simulink model "IEEE5BusSystemModel_std_UFLS"  (R2019b)
settings: Solver=ode4  StartTime=0.0  StopTime=300  MaxStep=1e-4  RelTol=1e-3
InitFcn:
  | startup_RTS
values from neighbouring files (symbols this model uses):
  C = b/(2*pi*60*Zn)    [startup_RTS.m]
  C0 = C/3    [startup_RTS.m]
  fn = 50    [startup_RTS.m]
  In = Sn/(sqrt(3)*Vn)    [startup_RTS.m]
  L = x*Zn/(2*pi*60)    [startup_RTS.m]
  L0 = 3*L    [startup_RTS.m]
  len = ceil(0.95*300000*T_prop)    [startup_RTS.m]
  PL1 = 300e6    (= 300000000)    [startup_RTS.m]
  PL2 = 300e6    (= 300000000)    [startup_RTS.m]
  PL3 = 300e6    (= 300000000)    [startup_RTS.m]
  QL1 = 30e6    (= 30000000)    [startup_RTS.m]
  QL2 = 30e6    (= 30000000)    [startup_RTS.m]
  QL3 = 30e6    (= 30000000)    [startup_RTS.m]
  R = r*Zn    [startup_RTS.m]
  R0 = 3*R    [startup_RTS.m]
  Sn = 1000e6    (= 1000000000)    [startup_RTS.m]
  t_cont = 100    [startup_RTS.m]
  Vn = 345e3    (= 345000)    [startup_RTS.m]
undefined symbols (not defined in the file or in its folder): D1, Delta
libraries: powerlib x42, powerlib_meascontrol x39, dspswit3 x10, dspstat3 x3, sps_avr x3, spsExcitationSystemModel x3
(part 3 of 7)

== system IEEE5BusSystemModel_std_UFLS/Subsystem2/PMU_e-IpDFT_P-class ==
  Uabc : Inport
  Constant1 : Constant  Value=dF  SampleTime=Ts_p
  Constant2 : Constant  Value=0  SampleTime=Ts_p
  Counter : dspswit3/Counter  Direction=Up  CountEvent=Free running  CounterSize=User defined  MaxCount=M-1  InitialCount=1  Output=Hit  HitValue=0  ResetInput=off  SamplesPerFrame=1  Ts=Ts_p  CntDtype=double  HitDtype=Logical
  Demux1 : Demux  Outputs=3
  Ia_est : Subsystem
  Terminator3 : Terminator
  Terminator4 : Terminator
  Frequency : Outport  VectorParamsAs1DForOutWhenUnconnected=off
  Amplitude : Outport  Port=2  VectorParamsAs1DForOutWhenUnconnected=off
  Phase : Outport  Port=3  VectorParamsAs1DForOutWhenUnconnected=off
  wires:
  Ia_est/1(Frequency) -> Frequency/1
  Ia_est/2(Amplitude) -> Amplitude/1
  Ia_est/3(Phase) -> Phase/1
  Uabc/1 -> Demux1/1
  Demux1/1 -> Ia_est/1(signal)
  Counter/1 -> Ia_est/2(Hit)
  Constant1/1 -> Ia_est/4(dF [Hz])
  Constant2/1 -> Ia_est/3(dT [s])
  Demux1/2 -> Terminator3/1
  Demux1/3 -> Terminator4/1

== system IEEE5BusSystemModel_std_UFLS/Subsystem2/PMU_e-IpDFT_P-class1 ==
  Uabc : Inport
  Constant1 : Constant  Value=dF  SampleTime=Ts_p
  Constant2 : Constant  Value=0  SampleTime=Ts_p
  Counter : dspswit3/Counter  Direction=Up  CountEvent=Free running  CounterSize=User defined  MaxCount=M-1  InitialCount=1  Output=Hit  HitValue=0  ResetInput=off  SamplesPerFrame=1  Ts=Ts_p  CntDtype=double  HitDtype=Logical
  Demux1 : Demux  Outputs=3
  Ia_est : Subsystem
  Terminator3 : Terminator
  Terminator4 : Terminator
  Frequency : Outport  VectorParamsAs1DForOutWhenUnconnected=off
  Amplitude : Outport  Port=2  VectorParamsAs1DForOutWhenUnconnected=off
  Phase : Outport  Port=3  VectorParamsAs1DForOutWhenUnconnected=off
  wires:
  Demux1/3 -> Terminator4/1
  Demux1/2 -> Terminator3/1
  Constant2/1 -> Ia_est/3(dT [s])
  Constant1/1 -> Ia_est/4(dF [Hz])
  Counter/1 -> Ia_est/2(Hit)
  Demux1/1 -> Ia_est/1(signal)
  Uabc/1 -> Demux1/1
  Ia_est/3(Phase) -> Phase/1
  Ia_est/2(Amplitude) -> Amplitude/1
  Ia_est/1(Frequency) -> Frequency/1

== system IEEE5BusSystemModel_std_UFLS/Subsystem3/PMU_e-IpDFT_P-class ==
  Uabc : Inport
  Constant1 : Constant  Value=dF  SampleTime=Ts_p
  Constant2 : Constant  Value=0  SampleTime=Ts_p
  Counter : dspswit3/Counter  Direction=Up  CountEvent=Free running  CounterSize=User defined  MaxCount=M-1  InitialCount=1  Output=Hit  HitValue=0  ResetInput=off  SamplesPerFrame=1  Ts=Ts_p  CntDtype=double  HitDtype=Logical
  Demux1 : Demux  Outputs=3
  Ia_est : Subsystem
  Terminator3 : Terminator
  Terminator4 : Terminator
  Frequency : Outport  VectorParamsAs1DForOutWhenUnconnected=off
  Amplitude : Outport  Port=2  VectorParamsAs1DForOutWhenUnconnected=off
  Phase : Outport  Port=3  VectorParamsAs1DForOutWhenUnconnected=off
  wires:
  Demux1/3 -> Terminator4/1
  Demux1/2 -> Terminator3/1
  Constant2/1 -> Ia_est/3(dT [s])
  Constant1/1 -> Ia_est/4(dF [Hz])
  Counter/1 -> Ia_est/2(Hit)
  Demux1/1 -> Ia_est/1(signal)
  Uabc/1 -> Demux1/1
  Ia_est/3(Phase) -> Phase/1
  Ia_est/2(Amplitude) -> Amplitude/1
  Ia_est/1(Frequency) -> Frequency/1

== system IEEE5BusSystemModel_std_UFLS/Subsystem3/PMU_e-IpDFT_P-class1 ==
  Uabc : Inport
  Constant1 : Constant  Value=dF  SampleTime=Ts_p
  Constant2 : Constant  Value=0  SampleTime=Ts_p
  Counter : dspswit3/Counter  Direction=Up  CountEvent=Free running  CounterSize=User defined  MaxCount=M-1  InitialCount=1  Output=Hit  HitValue=0  ResetInput=off  SamplesPerFrame=1  Ts=Ts_p  CntDtype=double  HitDtype=Logical
  Demux1 : Demux  Outputs=3
  Ia_est : Subsystem
  Terminator3 : Terminator
  Terminator4 : Terminator
  Frequency : Outport  VectorParamsAs1DForOutWhenUnconnected=off
  Amplitude : Outport  Port=2  VectorParamsAs1DForOutWhenUnconnected=off
  Phase : Outport  Port=3  VectorParamsAs1DForOutWhenUnconnected=off
  wires:
  Ia_est/1(Frequency) -> Frequency/1
  Ia_est/2(Amplitude) -> Amplitude/1
  Ia_est/3(Phase) -> Phase/1
  Uabc/1 -> Demux1/1
  Demux1/1 -> Ia_est/1(signal)
  Counter/1 -> Ia_est/2(Hit)
  Constant1/1 -> Ia_est/4(dF [Hz])
  Constant2/1 -> Ia_est/3(dT [s])
  Demux1/2 -> Terminator3/1
  Demux1/3 -> Terminator4/1

== system IEEE5BusSystemModel_std_UFLS/Subsystem4/PMU_e-IpDFT_P-class ==
  Uabc : Inport
  Constant1 : Constant  Value=dF  SampleTime=Ts_p
  Constant2 : Constant  Value=0  SampleTime=Ts_p
  Counter : dspswit3/Counter  Direction=Up  CountEvent=Free running  CounterSize=User defined  MaxCount=M-1  InitialCount=1  Output=Hit  HitValue=0  ResetInput=off  SamplesPerFrame=1  Ts=Ts_p  CntDtype=double  HitDtype=Logical
  Demux1 : Demux  Outputs=3
  Ia_est : Subsystem
  Terminator3 : Terminator
  Terminator4 : Terminator
  Frequency : Outport  VectorParamsAs1DForOutWhenUnconnected=off
  Amplitude : Outport  Port=2  VectorParamsAs1DForOutWhenUnconnected=off
  Phase : Outport  Port=3  VectorParamsAs1DForOutWhenUnconnected=off
  wires:
  Ia_est/1(Frequency) -> Frequency/1
  Ia_est/2(Amplitude) -> Amplitude/1
  Ia_est/3(Phase) -> Phase/1
  Uabc/1 -> Demux1/1
  Demux1/1 -> Ia_est/1(signal)
  Counter/1 -> Ia_est/2(Hit)
  Constant1/1 -> Ia_est/4(dF [Hz])
  Constant2/1 -> Ia_est/3(dT [s])
  Demux1/2 -> Terminator3/1
  Demux1/3 -> Terminator4/1

== system IEEE5BusSystemModel_std_UFLS/Subsystem4/PMU_e-IpDFT_P-class1 ==
  Uabc : Inport
  Constant1 : Constant  Value=dF  SampleTime=Ts_p
  Constant2 : Constant  Value=0  SampleTime=Ts_p
  Counter : dspswit3/Counter  Direction=Up  CountEvent=Free running  CounterSize=User defined  MaxCount=M-1  InitialCount=1  Output=Hit  HitValue=0  ResetInput=off  SamplesPerFrame=1  Ts=Ts_p  CntDtype=double  HitDtype=Logical
  Demux1 : Demux  Outputs=3
  Ia_est : Subsystem
  Terminator3 : Terminator
  Terminator4 : Terminator
  Frequency : Outport  VectorParamsAs1DForOutWhenUnconnected=off
  Amplitude : Outport  Port=2  VectorParamsAs1DForOutWhenUnconnected=off
  Phase : Outport  Port=3  VectorParamsAs1DForOutWhenUnconnected=off
  wires:
  Demux1/3 -> Terminator4/1
  Demux1/2 -> Terminator3/1
  Constant2/1 -> Ia_est/3(dT [s])
  Constant1/1 -> Ia_est/4(dF [Hz])
  Counter/1 -> Ia_est/2(Hit)
  Demux1/1 -> Ia_est/1(signal)
  Uabc/1 -> Demux1/1
  Ia_est/3(Phase) -> Phase/1
  Ia_est/2(Amplitude) -> Amplitude/1
  Ia_est/1(Frequency) -> Frequency/1

== system IEEE5BusSystemModel_std_UFLS/Subsystem5/PMU_e-IpDFT_P-class ==
  Uabc : Inport
  Constant1 : Constant  Value=dF  SampleTime=Ts_p
  Constant2 : Constant  Value=0  SampleTime=Ts_p
  Counter : dspswit3/Counter  Direction=Up  CountEvent=Free running  CounterSize=User defined  MaxCount=M-1  InitialCount=1  Output=Hit  HitValue=0  ResetInput=off  SamplesPerFrame=1  Ts=Ts_p  CntDtype=double  HitDtype=Logical
  Demux1 : Demux  Outputs=3
  Ia_est : Subsystem
  Terminator3 : Terminator
  Terminator4 : Terminator
  Frequency : Outport  VectorParamsAs1DForOutWhenUnconnected=off
  Amplitude : Outport  Port=2  VectorParamsAs1DForOutWhenUnconnected=off
  Phase : Outport  Port=3  VectorParamsAs1DForOutWhenUnconnected=off
  wires:
  Ia_est/1(Frequency) -> Frequency/1
  Ia_est/2(Amplitude) -> Amplitude/1
  Ia_est/3(Phase) -> Phase/1
  Uabc/1 -> Demux1/1
  Demux1/1 -> Ia_est/1(signal)
  Counter/1 -> Ia_est/2(Hit)
  Constant1/1 -> Ia_est/4(dF [Hz])
  Constant2/1 -> Ia_est/3(dT [s])
  Demux1/2 -> Terminator3/1
  Demux1/3 -> Terminator4/1

== system IEEE5BusSystemModel_std_UFLS/Subsystem5/PMU_e-IpDFT_P-class1 ==
  Uabc : Inport
  Constant1 : Constant  Value=dF  SampleTime=Ts_p
  Constant2 : Constant  Value=0  SampleTime=Ts_p
  Counter : dspswit3/Counter  Direction=Up  CountEvent=Free running  CounterSize=User defined  MaxCount=M-1  InitialCount=1  Output=Hit  HitValue=0  ResetInput=off  SamplesPerFrame=1  Ts=Ts_p  CntDtype=double  HitDtype=Logical
  Demux1 : Demux  Outputs=3
  Ia_est : Subsystem
  Terminator3 : Terminator
  Terminator4 : Terminator
  Frequency : Outport  VectorParamsAs1DForOutWhenUnconnected=off
  Amplitude : Outport  Port=2  VectorParamsAs1DForOutWhenUnconnected=off
  Phase : Outport  Port=3  VectorParamsAs1DForOutWhenUnconnected=off
  wires:
  Demux1/3 -> Terminator4/1
  Demux1/2 -> Terminator3/1
  Constant2/1 -> Ia_est/3(dT [s])
  Constant1/1 -> Ia_est/4(dF [Hz])
  Counter/1 -> Ia_est/2(Hit)
  Demux1/1 -> Ia_est/1(signal)
  Uabc/1 -> Demux1/1
  Ia_est/3(Phase) -> Phase/1
  Ia_est/2(Amplitude) -> Amplitude/1
  Ia_est/1(Frequency) -> Frequency/1

== system IEEE5BusSystemModel_std_UFLS/Dynamic Load/Load 8/Load shedding ==
  note: P=P0(V/V0) Kpv * [1+Kpf(f-f0)]
  note: Q=Q0(V/V0)[Kqv(1+Kqf(f-f0)]
  note: Q=Q0(V/V0)[Kqv(1+Kqf(f-f0)]
  note: P=P0(V/V0) Kpv * [1+Kpf(f-f0)]
  " f_PLL" : Inport
  Vamp_rms : Inport  Port=2
  load : Inport  Port=3
  Constant2 : Constant
  Constant3 : Constant  Value=50
  Constant4 : Constant
  Demux : Demux  Outputs=2
  Kpf : Gain
  Kpv : Constant  Value=1.4
  Kqf : Gain  Gain=-1.4
  Kqv : Constant  Value=1.5
  Math Function : Math  Operator=pow  SaturateOnIntegerOverflow=on
  Math Function1 : Math  Operator=pow  SaturateOnIntegerOverflow=on
  Mux : Mux  Inputs=2
  Product2 : Product  Inputs=3
  Product4 : Product  Inputs=3
  Saturation : Saturate  UpperLimit=1.2  LowerLimit=0
  Saturation1 : Saturate  UpperLimit=3/fn  LowerLimit=-3/fn
  Sum : Sum  Inputs=|++
  Sum1 : Sum  Inputs=|+-
  Sum2 : Sum  Inputs=|++
  V/V0 : Gain  Gain=sqrt(3)/345e3
  fpu : Gain  Gain=0.02
  Load Power : Outport  VectorParamsAs1DForOutWhenUnconnected=off
  wires:
  Product2/1 -> Mux/1
  Demux/1 -> Product2/1  "P0"
  Math Function/1 -> Product2/2
  Sum/1 -> Product2/3
  Constant2/1 -> Sum/1
  Constant3/1 -> Sum1/2
  Demux/2 -> Product4/1  "Q0"
  Math Function1/1 -> Product4/2
  Sum2/1 -> Product4/3
  Constant4/1 -> Sum2/1
  Sum1/1 -> fpu/1
  Product4/1 -> Mux/2
  Saturation1/1 -> Kpf/1, Kqf/1
  load/1 -> Demux/1
  fpu/1 -> Saturation1/1
  " f_PLL"/1 -> Sum1/1
  Vamp_rms/1 -> V/V0/1
  Mux/1 -> Load Power/1
  V/V0/1 -> Saturation/1  "Vamp-p"
  Saturation/1 -> Math Function/1, Math Function1/1
  Kpv/1 -> Math Function/2
  Kqv/1 -> Math Function1/2
  Kqf/1 -> Sum2/2
  Kpf/1 -> Sum/2

== system IEEE5BusSystemModel_std_UFLS/Dynamic Load1/Load 8/Load shedding ==
  note: P=P0(V/V0) Kpv * [1+Kpf(f-f0)]
  note: Q=Q0(V/V0)[Kqv(1+Kqf(f-f0)]
  note: Q=Q0(V/V0)[Kqv(1+Kqf(f-f0)]
  note: P=P0(V/V0) Kpv * [1+Kpf(f-f0)]
  " f_PLL" : Inport
  Vamp_rms : Inport  Port=2
  load : Inport  Port=3
  Constant2 : Constant
  Constant3 : Constant  Value=50
  Constant4 : Constant
  Demux : Demux  Outputs=2
  Kpf : Gain
  Kpv : Constant  Value=1.4
  Kqf : Gain  Gain=-1.6
  Kqv : Constant  Value=1.7
  Math Function : Math  Operator=pow  SaturateOnIntegerOverflow=on
  Math Function1 : Math  Operator=pow  SaturateOnIntegerOverflow=on
  Mux : Mux  Inputs=2
  Product2 : Product  Inputs=3
  Product4 : Product  Inputs=3
  Saturation : Saturate  UpperLimit=1.2  LowerLimit=0
  Saturation1 : Saturate  UpperLimit=3/fn  LowerLimit=-3/fn
  Sum : Sum  Inputs=|++
  Sum1 : Sum  Inputs=|+-
  Sum2 : Sum  Inputs=|++
  V/V0 : Gain  Gain=sqrt(3)/345e3
  fpu : Gain  Gain=0.02
  Load Power : Outport  VectorParamsAs1DForOutWhenUnconnected=off
  wires:
  Kpf/1 -> Sum/2
  Kqf/1 -> Sum2/2
  Kqv/1 -> Math Function1/2
  Kpv/1 -> Math Function/2
  Saturation/1 -> Math Function1/1, Math Function/1
  V/V0/1 -> Saturation/1  "Vamp-p"
  Mux/1 -> Load Power/1
  Vamp_rms/1 -> V/V0/1
  " f_PLL"/1 -> Sum1/1
  fpu/1 -> Saturation1/1
  load/1 -> Demux/1
  Saturation1/1 -> Kqf/1, Kpf/1
  Product4/1 -> Mux/2
  Sum1/1 -> fpu/1
  Constant4/1 -> Sum2/1
  Sum2/1 -> Product4/3
  Math Function1/1 -> Product4/2
  Demux/2 -> Product4/1  "Q0"
  Constant3/1 -> Sum1/2
  Constant2/1 -> Sum/1
  Sum/1 -> Product2/3
  Math Function/1 -> Product2/2
  Demux/1 -> Product2/1  "P0"
  Product2/1 -> Mux/1

== system IEEE5BusSystemModel_std_UFLS/Dynamic Load2/Load 8/Load shedding ==
  note: P=P0(V/V0) Kpv * [1+Kpf(f-f0)]
  note: Q=Q0(V/V0)[Kqv(1+Kqf(f-f0)]
  note: Q=Q0(V/V0)[Kqv(1+Kqf(f-f0)]
  note: P=P0(V/V0) Kpv * [1+Kpf(f-f0)]
  " f_PLL" : Inport
  Vamp_rms : Inport  Port=2
  load : Inport  Port=3
  Constant2 : Constant
  Constant3 : Constant  Value=50
  Constant4 : Constant
  Demux : Demux  Outputs=2
  Kpf : Gain
  Kpv : Constant  Value=1.5
  Kqf : Gain  Gain=-1.5
  Kqv : Constant  Value=1.9
  Math Function : Math  Operator=pow  SaturateOnIntegerOverflow=on
  Math Function1 : Math  Operator=pow  SaturateOnIntegerOverflow=on
  Mux : Mux  Inputs=2
  Product2 : Product  Inputs=3
  Product4 : Product  Inputs=3
  Saturation : Saturate  UpperLimit=1.2  LowerLimit=0
  Saturation1 : Saturate  UpperLimit=3/fn  LowerLimit=-3/fn
  Sum : Sum  Inputs=|++
  Sum1 : Sum  Inputs=|+-
  Sum2 : Sum  Inputs=|++
  V/V0 : Gain  Gain=sqrt(3)/345e3
  fpu : Gain  Gain=0.02
  Load Power : Outport  VectorParamsAs1DForOutWhenUnconnected=off
  wires:
  Product2/1 -> Mux/1
  Demux/1 -> Product2/1  "P0"
  Math Function/1 -> Product2/2
  Sum/1 -> Product2/3
  Constant2/1 -> Sum/1
  Constant3/1 -> Sum1/2
  Demux/2 -> Product4/1  "Q0"
  Math Function1/1 -> Product4/2
  Sum2/1 -> Product4/3
  Constant4/1 -> Sum2/1
  Sum1/1 -> fpu/1
  Product4/1 -> Mux/2
  Saturation1/1 -> Kpf/1, Kqf/1
  load/1 -> Demux/1
  fpu/1 -> Saturation1/1
  " f_PLL"/1 -> Sum1/1
  Vamp_rms/1 -> V/V0/1
  Mux/1 -> Load Power/1
  V/V0/1 -> Saturation/1  "Vamp-p"
  Saturation/1 -> Math Function/1, Math Function1/1
  Kpv/1 -> Math Function/2
  Kqv/1 -> Math Function1/2
  Kqf/1 -> Sum2/2
  Kpf/1 -> Sum/2

== system IEEE5BusSystemModel_std_UFLS/Subsystem1/PMU_e-IpDFT_P-class/Ia_est ==
  signal : Inport
  Hit : Inport  Port=2
  dT [s] : Inport  Port=3
  dF [Hz] : Inport  Port=4
  Synchrophasor estimation : Subsystem
  mSDFT : Subsystem
  Frequency : Outport  VectorParamsAs1DForOutWhenUnconnected=off
  Amplitude : Outport  Port=2  VectorParamsAs1DForOutWhenUnconnected=off
  Phase : Outport  Port=3  VectorParamsAs1DForOutWhenUnconnected=off
  wires:
  dT [s]/1 -> Synchrophasor estimation/2(dT [s])
  Hit/1 -> mSDFT/2(Hit)
  Synchrophasor estimation/3(Phase) -> Phase/1
  Synchrophasor estimation/2(Amplitude) -> Amplitude/1
  mSDFT/1(DFT) -> Synchrophasor estimation/1(DFT)
  signal/1 -> mSDFT/1(signal)
  Synchrophasor estimation/1(Frequency) -> Frequency/1
  dF [Hz]/1 -> Synchrophasor estimation/3(dF [Hz])

== system IEEE5BusSystemModel_std_UFLS/Subsystem1/PMU_e-IpDFT_P-class1/Ia_est ==
  signal : Inport
  Hit : Inport  Port=2
  dT [s] : Inport  Port=3
  dF [Hz] : Inport  Port=4
  Synchrophasor estimation : Subsystem
  mSDFT : Subsystem
  Frequency : Outport  VectorParamsAs1DForOutWhenUnconnected=off
  Amplitude : Outport  Port=2  VectorParamsAs1DForOutWhenUnconnected=off
  Phase : Outport  Port=3  VectorParamsAs1DForOutWhenUnconnected=off
  wires:
  dF [Hz]/1 -> Synchrophasor estimation/3(dF [Hz])
  Synchrophasor estimation/1(Frequency) -> Frequency/1
  signal/1 -> mSDFT/1(signal)
  mSDFT/1(DFT) -> Synchrophasor estimation/1(DFT)
  Synchrophasor estimation/2(Amplitude) -> Amplitude/1
  Synchrophasor estimation/3(Phase) -> Phase/1
  Hit/1 -> mSDFT/2(Hit)
  dT [s]/1 -> Synchrophasor estimation/2(dT [s])

== system IEEE5BusSystemModel_std_UFLS/Subsystem2/PMU_e-IpDFT_P-class/Ia_est ==
  signal : Inport
  Hit : Inport  Port=2
  dT [s] : Inport  Port=3
  dF [Hz] : Inport  Port=4
  Synchrophasor estimation : Subsystem
  mSDFT : Subsystem
  Frequency : Outport  VectorParamsAs1DForOutWhenUnconnected=off
  Amplitude : Outport  Port=2  VectorParamsAs1DForOutWhenUnconnected=off
  Phase : Outport  Port=3  VectorParamsAs1DForOutWhenUnconnected=off
  wires:
  dF [Hz]/1 -> Synchrophasor estimation/3(dF [Hz])
  Synchrophasor estimation/1(Frequency) -> Frequency/1
  signal/1 -> mSDFT/1(signal)
  mSDFT/1(DFT) -> Synchrophasor estimation/1(DFT)
  Synchrophasor estimation/2(Amplitude) -> Amplitude/1
  Synchrophasor estimation/3(Phase) -> Phase/1
  Hit/1 -> mSDFT/2(Hit)
  dT [s]/1 -> Synchrophasor estimation/2(dT [s])

== system IEEE5BusSystemModel_std_UFLS/Subsystem2/PMU_e-IpDFT_P-class1/Ia_est ==
  signal : Inport
  Hit : Inport  Port=2
  dT [s] : Inport  Port=3
  dF [Hz] : Inport  Port=4
  Synchrophasor estimation : Subsystem
  mSDFT : Subsystem
  Frequency : Outport  VectorParamsAs1DForOutWhenUnconnected=off
  Amplitude : Outport  Port=2  VectorParamsAs1DForOutWhenUnconnected=off
  Phase : Outport  Port=3  VectorParamsAs1DForOutWhenUnconnected=off
  wires:
  dT [s]/1 -> Synchrophasor estimation/2(dT [s])
  Hit/1 -> mSDFT/2(Hit)
  Synchrophasor estimation/3(Phase) -> Phase/1
  Synchrophasor estimation/2(Amplitude) -> Amplitude/1
  mSDFT/1(DFT) -> Synchrophasor estimation/1(DFT)
  signal/1 -> mSDFT/1(signal)
  Synchrophasor estimation/1(Frequency) -> Frequency/1
  dF [Hz]/1 -> Synchrophasor estimation/3(dF [Hz])

== system IEEE5BusSystemModel_std_UFLS/Subsystem3/PMU_e-IpDFT_P-class/Ia_est ==
  signal : Inport
  Hit : Inport  Port=2
  dT [s] : Inport  Port=3
  dF [Hz] : Inport  Port=4
  Synchrophasor estimation : Subsystem
  mSDFT : Subsystem
  Frequency : Outport  VectorParamsAs1DForOutWhenUnconnected=off
  Amplitude : Outport  Port=2  VectorParamsAs1DForOutWhenUnconnected=off
  Phase : Outport  Port=3  VectorParamsAs1DForOutWhenUnconnected=off
  wires:
  dT [s]/1 -> Synchrophasor estimation/2(dT [s])
  Hit/1 -> mSDFT/2(Hit)
  Synchrophasor estimation/3(Phase) -> Phase/1
  Synchrophasor estimation/2(Amplitude) -> Amplitude/1
  mSDFT/1(DFT) -> Synchrophasor estimation/1(DFT)
  signal/1 -> mSDFT/1(signal)
  Synchrophasor estimation/1(Frequency) -> Frequency/1
  dF [Hz]/1 -> Synchrophasor estimation/3(dF [Hz])

== system IEEE5BusSystemModel_std_UFLS/Subsystem3/PMU_e-IpDFT_P-class1/Ia_est ==
  signal : Inport
  Hit : Inport  Port=2
  dT [s] : Inport  Port=3
  dF [Hz] : Inport  Port=4
  Synchrophasor estimation : Subsystem
  mSDFT : Subsystem
  Frequency : Outport  VectorParamsAs1DForOutWhenUnconnected=off
  Amplitude : Outport  Port=2  VectorParamsAs1DForOutWhenUnconnected=off
  Phase : Outport  Port=3  VectorParamsAs1DForOutWhenUnconnected=off
  wires:
  dF [Hz]/1 -> Synchrophasor estimation/3(dF [Hz])
  Synchrophasor estimation/1(Frequency) -> Frequency/1
  signal/1 -> mSDFT/1(signal)
  mSDFT/1(DFT) -> Synchrophasor estimation/1(DFT)
  Synchrophasor estimation/2(Amplitude) -> Amplitude/1
  Synchrophasor estimation/3(Phase) -> Phase/1
  Hit/1 -> mSDFT/2(Hit)
  dT [s]/1 -> Synchrophasor estimation/2(dT [s])

== system IEEE5BusSystemModel_std_UFLS/Subsystem4/PMU_e-IpDFT_P-class/Ia_est ==
  signal : Inport
  Hit : Inport  Port=2
  dT [s] : Inport  Port=3
  dF [Hz] : Inport  Port=4
  Synchrophasor estimation : Subsystem
  mSDFT : Subsystem
  Frequency : Outport  VectorParamsAs1DForOutWhenUnconnected=off
  Amplitude : Outport  Port=2  VectorParamsAs1DForOutWhenUnconnected=off
  Phase : Outport  Port=3  VectorParamsAs1DForOutWhenUnconnected=off
  wires:
  dF [Hz]/1 -> Synchrophasor estimation/3(dF [Hz])
  Synchrophasor estimation/1(Frequency) -> Frequency/1
  signal/1 -> mSDFT/1(signal)
  mSDFT/1(DFT) -> Synchrophasor estimation/1(DFT)
  Synchrophasor estimation/2(Amplitude) -> Amplitude/1
  Synchrophasor estimation/3(Phase) -> Phase/1
  Hit/1 -> mSDFT/2(Hit)
  dT [s]/1 -> Synchrophasor estimation/2(dT [s])

== system IEEE5BusSystemModel_std_UFLS/Subsystem4/PMU_e-IpDFT_P-class1/Ia_est ==
  signal : Inport
  Hit : Inport  Port=2
  dT [s] : Inport  Port=3
  dF [Hz] : Inport  Port=4
  Synchrophasor estimation : Subsystem
  mSDFT : Subsystem
  Frequency : Outport  VectorParamsAs1DForOutWhenUnconnected=off
  Amplitude : Outport  Port=2  VectorParamsAs1DForOutWhenUnconnected=off
  Phase : Outport  Port=3  VectorParamsAs1DForOutWhenUnconnected=off
  wires:
  dT [s]/1 -> Synchrophasor estimation/2(dT [s])
  Hit/1 -> mSDFT/2(Hit)
  Synchrophasor estimation/3(Phase) -> Phase/1
  Synchrophasor estimation/2(Amplitude) -> Amplitude/1
  mSDFT/1(DFT) -> Synchrophasor estimation/1(DFT)
  signal/1 -> mSDFT/1(signal)
  Synchrophasor estimation/1(Frequency) -> Frequency/1
  dF [Hz]/1 -> Synchrophasor estimation/3(dF [Hz])

== system IEEE5BusSystemModel_std_UFLS/Subsystem5/PMU_e-IpDFT_P-class/Ia_est ==
  signal : Inport
  Hit : Inport  Port=2
  dT [s] : Inport  Port=3
  dF [Hz] : Inport  Port=4
  Synchrophasor estimation : Subsystem
  mSDFT : Subsystem
  Frequency : Outport  VectorParamsAs1DForOutWhenUnconnected=off
  Amplitude : Outport  Port=2  VectorParamsAs1DForOutWhenUnconnected=off
  Phase : Outport  Port=3  VectorParamsAs1DForOutWhenUnconnected=off
  wires:
  dF [Hz]/1 -> Synchrophasor estimation/3(dF [Hz])
  Synchrophasor estimation/1(Frequency) -> Frequency/1
  signal/1 -> mSDFT/1(signal)
  mSDFT/1(DFT) -> Synchrophasor estimation/1(DFT)
  Synchrophasor estimation/2(Amplitude) -> Amplitude/1
  Synchrophasor estimation/3(Phase) -> Phase/1
  Hit/1 -> mSDFT/2(Hit)
  dT [s]/1 -> Synchrophasor estimation/2(dT [s])

== system IEEE5BusSystemModel_std_UFLS/Subsystem5/PMU_e-IpDFT_P-class1/Ia_est ==
  signal : Inport
  Hit : Inport  Port=2
  dT [s] : Inport  Port=3
  dF [Hz] : Inport  Port=4
  Synchrophasor estimation : Subsystem
  mSDFT : Subsystem
  Frequency : Outport  VectorParamsAs1DForOutWhenUnconnected=off
  Amplitude : Outport  Port=2  VectorParamsAs1DForOutWhenUnconnected=off
  Phase : Outport  Port=3  VectorParamsAs1DForOutWhenUnconnected=off
  wires:
  dT [s]/1 -> Synchrophasor estimation/2(dT [s])
  Hit/1 -> mSDFT/2(Hit)
  Synchrophasor estimation/3(Phase) -> Phase/1
  Synchrophasor estimation/2(Amplitude) -> Amplitude/1
  mSDFT/1(DFT) -> Synchrophasor estimation/1(DFT)
  signal/1 -> mSDFT/1(signal)
  Synchrophasor estimation/1(Frequency) -> Frequency/1
  dF [Hz]/1 -> Synchrophasor estimation/3(dF [Hz])

== system IEEE5BusSystemModel_std_UFLS/Subsystem1/PMU_e-IpDFT_P-class/Ia_est/Synchrophasor estimation ==
  DFT : Inport
  dT [s] : Inport  Port=2
  dF [Hz] : Inport  Port=3
  Amplitude - 1 : Subsystem
  Amplitude - 2 : Subsystem
  Complex to Magnitude-Angle1 : ComplexToMagnitudeAngle
  Complex to Magnitude-Angle2 : ComplexToMagnitudeAngle
  Demux1 : Demux  Outputs=5
  Frequency - 2 : Subsystem
  Hanning(Kmax) : Subsystem
  Hanning(Kmax+1) : Subsystem
  Hanning(Kmax-1) : Subsystem
  Phase - 2 : Subsystem
  Terminator : Terminator
  Terminator1 : Terminator
  "delta - 1 " : Subsystem
  delta - 2 : Subsystem
  epsilon : Subsystem
  spectral leakage compensation : Subsystem
  Frequency : Outport  VectorParamsAs1DForOutWhenUnconnected=off
  Amplitude : Outport  Port=2  VectorParamsAs1DForOutWhenUnconnected=off
  Phase : Outport  Port=3  VectorParamsAs1DForOutWhenUnconnected=off
  wires:
  DFT/1 -> Demux1/1
  Frequency - 2/1(frequency) -> Phase - 2/3(freq), Frequency/1
  Amplitude - 2/1(amplitude) -> Amplitude/1
  Demux1/5 -> Hanning(Kmax+1)/3(Kmax+2)
  Demux1/1 -> Hanning(Kmax-1)/1(Kmax-2)
  Demux1/2 -> Hanning(Kmax)/1(Kmax-1), Hanning(Kmax-1)/2(Kmax-1)
  Demux1/3 -> Hanning(Kmax-1)/3(Kmax), Hanning(Kmax+1)/1(Kmax), Hanning(Kmax)/2(Kmax)
  Demux1/4 -> Hanning(Kmax+1)/2(Kmax+1), Hanning(Kmax)/3(Kmax+1)
  Hanning(Kmax+1)/1(Hanning out) -> epsilon/2(X (k max+1))
  Hanning(Kmax)/1(Hanning out) -> "delta - 1 "/1(X (k max)), Amplitude - 1/2((X k_max)), spectral leakage compensation/4(X (k max))
  epsilon/1(X (Kmax + epsilon)) -> "delta - 1 "/2(X (k max + epsilon)), spectral leakage compensation/3(X (k max + epsilon))
  epsilon/2(epsilon) -> spectral leakage compensation/5(epsilon), delta - 2/3(epsilon), "delta - 1 "/3(epsilon)
  "delta - 1 "/1(delta) -> spectral leakage compensation/2(delta), Amplitude - 1/1(delta)
  spectral leakage compensation/1(X(k max)) -> delta - 2/1(X (k max)), Complex to Magnitude-Angle2/1, Amplitude - 2/2((X k_max))
  spectral leakage compensation/2(X(k max+epsilon)) -> delta - 2/2(X (k max + epsilon))
  delta - 2/1(delta) -> Frequency - 2/1(delta), Phase - 2/2(delta), Amplitude - 2/1(delta)
  Phase - 2/1(phase) -> Phase/1
  Complex to Magnitude-Angle1/2 -> spectral leakage compensation/6(ph X(k-1))
  Complex to Magnitude-Angle1/1 -> Terminator/1
  Complex to Magnitude-Angle2/2 -> Phase - 2/1(X k_max phase)
  Complex to Magnitude-Angle2/1 -> Terminator1/1
  dT [s]/1 -> Phase - 2/4(dT [s])
  Amplitude - 1/1(amplitude) -> spectral leakage compensation/1(Amplitude)
  Hanning(Kmax-1)/1(Hanning out) -> Complex to Magnitude-Angle1/1, epsilon/1(X (k max -1))
  dF [Hz]/1 -> Frequency - 2/2(dF [Hz])

== system IEEE5BusSystemModel_std_UFLS/Subsystem1/PMU_e-IpDFT_P-class/Ia_est/mSDFT ==
  signal : Inport
  Hit : Inport  Port=2
  Delay_M : Delay  DelayLength=M  SampleTime=Ts_p
  Kmax : Subsystem
  Kmax+1 : Subsystem
  Kmax+2 : Subsystem
  Kmax-1 : Subsystem
  Kmax-2 : Subsystem
  Mux : Mux  Inputs=5
  DFT : Outport  VectorParamsAs1DForOutWhenUnconnected=off
  wires:
  Mux/1 -> DFT/1
  Kmax+2/1(X(k)) -> Mux/5
  Kmax+1/1(X(k)) -> Mux/4
  Kmax/1(X(k)) -> Mux/3
  Kmax-1/1(X(k)) -> Mux/2
  Kmax-2/1(X(k)) -> Mux/1
  signal/1 -> Kmax-2/1(x(n)), Kmax-1/1(x(n)), Kmax+2/1(x(n)), Kmax+1/1(x(n)), Kmax/1(x(n)), Delay_M/1
  Delay_M/1 -> Kmax/2(x(n-M)), Kmax+1/2(x(n-M)), Kmax+2/2(x(n-M)), Kmax-1/2(x(n-M)), Kmax-2/2(x(n-M))
  Hit/1 -> Kmax-2/3(trigger), Kmax-1/3(trigger), Kmax/3(trigger), Kmax+1/3(trigger), Kmax+2/3(trigger)

== system IEEE5BusSystemModel_std_UFLS/Subsystem1/PMU_e-IpDFT_P-class1/Ia_est/Synchrophasor estimation ==
  DFT : Inport
  dT [s] : Inport  Port=2
  dF [Hz] : Inport  Port=3
  Amplitude - 1 : Subsystem
  Amplitude - 2 : Subsystem
  Complex to Magnitude-Angle1 : ComplexToMagnitudeAngle
  Complex to Magnitude-Angle2 : ComplexToMagnitudeAngle
  Demux1 : Demux  Outputs=5
  Frequency - 2 : Subsystem
  Hanning(Kmax) : Subsystem
  Hanning(Kmax+1) : Subsystem
  Hanning(Kmax-1) : Subsystem
  Phase - 2 : Subsystem
  Terminator : Terminator
  Terminator1 : Terminator
  "delta - 1 " : Subsystem
  delta - 2 : Subsystem
  epsilon : Subsystem
  spectral leakage compensation : Subsystem
  Frequency : Outport  VectorParamsAs1DForOutWhenUnconnected=off
  Amplitude : Outport  Port=2  VectorParamsAs1DForOutWhenUnconnected=off
  Phase : Outport  Port=3  VectorParamsAs1DForOutWhenUnconnected=off
  wires:
  dF [Hz]/1 -> Frequency - 2/2(dF [Hz])
  Hanning(Kmax-1)/1(Hanning out) -> epsilon/1(X (k max -1)), Complex to Magnitude-Angle1/1
  Amplitude - 1/1(amplitude) -> spectral leakage compensation/1(Amplitude)
  dT [s]/1 -> Phase - 2/4(dT [s])
  Complex to Magnitude-Angle2/1 -> Terminator1/1
  Complex to Magnitude-Angle2/2 -> Phase - 2/1(X k_max phase)
  Complex to Magnitude-Angle1/1 -> Terminator/1
  Complex to Magnitude-Angle1/2 -> spectral leakage compensation/6(ph X(k-1))
  Phase - 2/1(phase) -> Phase/1
  delta - 2/1(delta) -> Amplitude - 2/1(delta), Phase - 2/2(delta), Frequency - 2/1(delta)
  spectral leakage compensation/2(X(k max+epsilon)) -> delta - 2/2(X (k max + epsilon))
  spectral leakage compensation/1(X(k max)) -> Amplitude - 2/2((X k_max)), Complex to Magnitude-Angle2/1, delta - 2/1(X (k max))
  "delta - 1 "/1(delta) -> Amplitude - 1/1(delta), spectral leakage compensation/2(delta)
  epsilon/2(epsilon) -> "delta - 1 "/3(epsilon), delta - 2/3(epsilon), spectral leakage compensation/5(epsilon)
  epsilon/1(X (Kmax + epsilon)) -> spectral leakage compensation/3(X (k max + epsilon)), "delta - 1 "/2(X (k max + epsilon))
  Hanning(Kmax)/1(Hanning out) -> spectral leakage compensation/4(X (k max)), Amplitude - 1/2((X k_max)), "delta - 1 "/1(X (k max))
  Hanning(Kmax+1)/1(Hanning out) -> epsilon/2(X (k max+1))
  Demux1/4 -> Hanning(Kmax)/3(Kmax+1), Hanning(Kmax+1)/2(Kmax+1)
  Demux1/3 -> Hanning(Kmax)/2(Kmax), Hanning(Kmax+1)/1(Kmax), Hanning(Kmax-1)/3(Kmax)
  Demux1/2 -> Hanning(Kmax-1)/2(Kmax-1), Hanning(Kmax)/1(Kmax-1)
  Demux1/1 -> Hanning(Kmax-1)/1(Kmax-2)
  Demux1/5 -> Hanning(Kmax+1)/3(Kmax+2)
  Amplitude - 2/1(amplitude) -> Amplitude/1
  Frequency - 2/1(frequency) -> Frequency/1, Phase - 2/3(freq)
  DFT/1 -> Demux1/1

== system IEEE5BusSystemModel_std_UFLS/Subsystem1/PMU_e-IpDFT_P-class1/Ia_est/mSDFT ==
  signal : Inport
  Hit : Inport  Port=2
  Delay_M : Delay  DelayLength=M  SampleTime=Ts_p
  Kmax : Subsystem
  Kmax+1 : Subsystem
  Kmax+2 : Subsystem
  Kmax-1 : Subsystem
  Kmax-2 : Subsystem
  Mux : Mux  Inputs=5
  DFT : Outport  VectorParamsAs1DForOutWhenUnconnected=off
  wires:
  Hit/1 -> Kmax+2/3(trigger), Kmax+1/3(trigger), Kmax/3(trigger), Kmax-1/3(trigger), Kmax-2/3(trigger)
  Delay_M/1 -> Kmax-2/2(x(n-M)), Kmax-1/2(x(n-M)), Kmax+2/2(x(n-M)), Kmax+1/2(x(n-M)), Kmax/2(x(n-M))
  signal/1 -> Delay_M/1, Kmax/1(x(n)), Kmax+1/1(x(n)), Kmax+2/1(x(n)), Kmax-1/1(x(n)), Kmax-2/1(x(n))
  Kmax-2/1(X(k)) -> Mux/1
  Kmax-1/1(X(k)) -> Mux/2
  Kmax/1(X(k)) -> Mux/3
  Kmax+1/1(X(k)) -> Mux/4
  Kmax+2/1(X(k)) -> Mux/5
  Mux/1 -> DFT/1

== system IEEE5BusSystemModel_std_UFLS/Subsystem2/PMU_e-IpDFT_P-class/Ia_est/Synchrophasor estimation ==
  DFT : Inport
  dT [s] : Inport  Port=2
  dF [Hz] : Inport  Port=3
  Amplitude - 1 : Subsystem
  Amplitude - 2 : Subsystem
  Complex to Magnitude-Angle1 : ComplexToMagnitudeAngle
  Complex to Magnitude-Angle2 : ComplexToMagnitudeAngle
  Demux1 : Demux  Outputs=5
  Frequency - 2 : Subsystem
  Hanning(Kmax) : Subsystem
  Hanning(Kmax+1) : Subsystem
  Hanning(Kmax-1) : Subsystem
  Phase - 2 : Subsystem
  Terminator : Terminator
  Terminator1 : Terminator
  "delta - 1 " : Subsystem
  delta - 2 : Subsystem
  epsilon : Subsystem
  spectral leakage compensation : Subsystem
  Frequency : Outport  VectorParamsAs1DForOutWhenUnconnected=off
  Amplitude : Outport  Port=2  VectorParamsAs1DForOutWhenUnconnected=off
  Phase : Outport  Port=3  VectorParamsAs1DForOutWhenUnconnected=off
  wires:
  dF [Hz]/1 -> Frequency - 2/2(dF [Hz])
  Hanning(Kmax-1)/1(Hanning out) -> epsilon/1(X (k max -1)), Complex to Magnitude-Angle1/1
  Amplitude - 1/1(amplitude) -> spectral leakage compensation/1(Amplitude)
  dT [s]/1 -> Phase - 2/4(dT [s])
  Complex to Magnitude-Angle2/1 -> Terminator1/1
  Complex to Magnitude-Angle2/2 -> Phase - 2/1(X k_max phase)
  Complex to Magnitude-Angle1/1 -> Terminator/1
  Complex to Magnitude-Angle1/2 -> spectral leakage compensation/6(ph X(k-1))
  Phase - 2/1(phase) -> Phase/1
  delta - 2/1(delta) -> Amplitude - 2/1(delta), Phase - 2/2(delta), Frequency - 2/1(delta)
  spectral leakage compensation/2(X(k max+epsilon)) -> delta - 2/2(X (k max + epsilon))
  spectral leakage compensation/1(X(k max)) -> Amplitude - 2/2((X k_max)), Complex to Magnitude-Angle2/1, delta - 2/1(X (k max))
  "delta - 1 "/1(delta) -> Amplitude - 1/1(delta), spectral leakage compensation/2(delta)
  epsilon/2(epsilon) -> "delta - 1 "/3(epsilon), delta - 2/3(epsilon), spectral leakage compensation/5(epsilon)
  epsilon/1(X (Kmax + epsilon)) -> spectral leakage compensation/3(X (k max + epsilon)), "delta - 1 "/2(X (k max + epsilon))
  Hanning(Kmax)/1(Hanning out) -> spectral leakage compensation/4(X (k max)), Amplitude - 1/2((X k_max)), "delta - 1 "/1(X (k max))
  Hanning(Kmax+1)/1(Hanning out) -> epsilon/2(X (k max+1))
  Demux1/4 -> Hanning(Kmax)/3(Kmax+1), Hanning(Kmax+1)/2(Kmax+1)
  Demux1/3 -> Hanning(Kmax)/2(Kmax), Hanning(Kmax+1)/1(Kmax), Hanning(Kmax-1)/3(Kmax)
  Demux1/2 -> Hanning(Kmax-1)/2(Kmax-1), Hanning(Kmax)/1(Kmax-1)
  Demux1/1 -> Hanning(Kmax-1)/1(Kmax-2)
  Demux1/5 -> Hanning(Kmax+1)/3(Kmax+2)
  Amplitude - 2/1(amplitude) -> Amplitude/1
  Frequency - 2/1(frequency) -> Frequency/1, Phase - 2/3(freq)
  DFT/1 -> Demux1/1

== system IEEE5BusSystemModel_std_UFLS/Subsystem2/PMU_e-IpDFT_P-class/Ia_est/mSDFT ==
  signal : Inport
  Hit : Inport  Port=2
  Delay_M : Delay  DelayLength=M  SampleTime=Ts_p
  Kmax : Subsystem
  Kmax+1 : Subsystem
  Kmax+2 : Subsystem
  Kmax-1 : Subsystem
  Kmax-2 : Subsystem
  Mux : Mux  Inputs=5
  DFT : Outport  VectorParamsAs1DForOutWhenUnconnected=off
  wires:
  Hit/1 -> Kmax+2/3(trigger), Kmax+1/3(trigger), Kmax/3(trigger), Kmax-1/3(trigger), Kmax-2/3(trigger)
  Delay_M/1 -> Kmax-2/2(x(n-M)), Kmax-1/2(x(n-M)), Kmax+2/2(x(n-M)), Kmax+1/2(x(n-M)), Kmax/2(x(n-M))
  signal/1 -> Delay_M/1, Kmax/1(x(n)), Kmax+1/1(x(n)), Kmax+2/1(x(n)), Kmax-1/1(x(n)), Kmax-2/1(x(n))
  Kmax-2/1(X(k)) -> Mux/1
  Kmax-1/1(X(k)) -> Mux/2
  Kmax/1(X(k)) -> Mux/3
  Kmax+1/1(X(k)) -> Mux/4
  Kmax+2/1(X(k)) -> Mux/5
  Mux/1 -> DFT/1

== system IEEE5BusSystemModel_std_UFLS/Subsystem2/PMU_e-IpDFT_P-class1/Ia_est/Synchrophasor estimation ==
  DFT : Inport
  dT [s] : Inport  Port=2
  dF [Hz] : Inport  Port=3
  Amplitude - 1 : Subsystem
  Amplitude - 2 : Subsystem
  Complex to Magnitude-Angle1 : ComplexToMagnitudeAngle
  Complex to Magnitude-Angle2 : ComplexToMagnitudeAngle
  Demux1 : Demux  Outputs=5
  Frequency - 2 : Subsystem
  Hanning(Kmax) : Subsystem
  Hanning(Kmax+1) : Subsystem
  Hanning(Kmax-1) : Subsystem
  Phase - 2 : Subsystem
  Terminator : Terminator
  Terminator1 : Terminator
  "delta - 1 " : Subsystem
  delta - 2 : Subsystem
  epsilon : Subsystem
  spectral leakage compensation : Subsystem
  Frequency : Outport  VectorParamsAs1DForOutWhenUnconnected=off
  Amplitude : Outport  Port=2  VectorParamsAs1DForOutWhenUnconnected=off
  Phase : Outport  Port=3  VectorParamsAs1DForOutWhenUnconnected=off
  wires:
  DFT/1 -> Demux1/1
  Frequency - 2/1(frequency) -> Phase - 2/3(freq), Frequency/1
  Amplitude - 2/1(amplitude) -> Amplitude/1
  Demux1/5 -> Hanning(Kmax+1)/3(Kmax+2)
  Demux1/1 -> Hanning(Kmax-1)/1(Kmax-2)
  Demux1/2 -> Hanning(Kmax)/1(Kmax-1), Hanning(Kmax-1)/2(Kmax-1)
  Demux1/3 -> Hanning(Kmax-1)/3(Kmax), Hanning(Kmax+1)/1(Kmax), Hanning(Kmax)/2(Kmax)
  Demux1/4 -> Hanning(Kmax+1)/2(Kmax+1), Hanning(Kmax)/3(Kmax+1)
  Hanning(Kmax+1)/1(Hanning out) -> epsilon/2(X (k max+1))
  Hanning(Kmax)/1(Hanning out) -> "delta - 1 "/1(X (k max)), Amplitude - 1/2((X k_max)), spectral leakage compensation/4(X (k max))
  epsilon/1(X (Kmax + epsilon)) -> "delta - 1 "/2(X (k max + epsilon)), spectral leakage compensation/3(X (k max + epsilon))
  epsilon/2(epsilon) -> spectral leakage compensation/5(epsilon), delta - 2/3(epsilon), "delta - 1 "/3(epsilon)
  "delta - 1 "/1(delta) -> spectral leakage compensation/2(delta), Amplitude - 1/1(delta)
  spectral leakage compensation/1(X(k max)) -> delta - 2/1(X (k max)), Complex to Magnitude-Angle2/1, Amplitude - 2/2((X k_max))
  spectral leakage compensation/2(X(k max+epsilon)) -> delta - 2/2(X (k max + epsilon))
  delta - 2/1(delta) -> Frequency - 2/1(delta), Phase - 2/2(delta), Amplitude - 2/1(delta)
  Phase - 2/1(phase) -> Phase/1
  Complex to Magnitude-Angle1/2 -> spectral leakage compensation/6(ph X(k-1))
  Complex to Magnitude-Angle1/1 -> Terminator/1
  Complex to Magnitude-Angle2/2 -> Phase - 2/1(X k_max phase)
  Complex to Magnitude-Angle2/1 -> Terminator1/1
  dT [s]/1 -> Phase - 2/4(dT [s])
  Amplitude - 1/1(amplitude) -> spectral leakage compensation/1(Amplitude)
  Hanning(Kmax-1)/1(Hanning out) -> Complex to Magnitude-Angle1/1, epsilon/1(X (k max -1))
  dF [Hz]/1 -> Frequency - 2/2(dF [Hz])

== system IEEE5BusSystemModel_std_UFLS/Subsystem2/PMU_e-IpDFT_P-class1/Ia_est/mSDFT ==
  signal : Inport
  Hit : Inport  Port=2
  Delay_M : Delay  DelayLength=M  SampleTime=Ts_p
  Kmax : Subsystem
  Kmax+1 : Subsystem
  Kmax+2 : Subsystem
  Kmax-1 : Subsystem
  Kmax-2 : Subsystem
  Mux : Mux  Inputs=5
  DFT : Outport  VectorParamsAs1DForOutWhenUnconnected=off
  wires:
  Mux/1 -> DFT/1
  Kmax+2/1(X(k)) -> Mux/5
  Kmax+1/1(X(k)) -> Mux/4
  Kmax/1(X(k)) -> Mux/3
  Kmax-1/1(X(k)) -> Mux/2
  Kmax-2/1(X(k)) -> Mux/1
  signal/1 -> Kmax-2/1(x(n)), Kmax-1/1(x(n)), Kmax+2/1(x(n)), Kmax+1/1(x(n)), Kmax/1(x(n)), Delay_M/1
  Delay_M/1 -> Kmax/2(x(n-M)), Kmax+1/2(x(n-M)), Kmax+2/2(x(n-M)), Kmax-1/2(x(n-M)), Kmax-2/2(x(n-M))
  Hit/1 -> Kmax-2/3(trigger), Kmax-1/3(trigger), Kmax/3(trigger), Kmax+1/3(trigger), Kmax+2/3(trigger)

== system IEEE5BusSystemModel_std_UFLS/Subsystem3/PMU_e-IpDFT_P-class/Ia_est/Synchrophasor estimation ==
  DFT : Inport
  dT [s] : Inport  Port=2
  dF [Hz] : Inport  Port=3
  Amplitude - 1 : Subsystem
  Amplitude - 2 : Subsystem
  Complex to Magnitude-Angle1 : ComplexToMagnitudeAngle
  Complex to Magnitude-Angle2 : ComplexToMagnitudeAngle
  Demux1 : Demux  Outputs=5
  Frequency - 2 : Subsystem
  Hanning(Kmax) : Subsystem
  Hanning(Kmax+1) : Subsystem
  Hanning(Kmax-1) : Subsystem
  Phase - 2 : Subsystem
  Terminator : Terminator
  Terminator1 : Terminator
  "delta - 1 " : Subsystem
  delta - 2 : Subsystem
  epsilon : Subsystem
  spectral leakage compensation : Subsystem
  Frequency : Outport  VectorParamsAs1DForOutWhenUnconnected=off
  Amplitude : Outport  Port=2  VectorParamsAs1DForOutWhenUnconnected=off
  Phase : Outport  Port=3  VectorParamsAs1DForOutWhenUnconnected=off
  wires:
  DFT/1 -> Demux1/1
  Frequency - 2/1(frequency) -> Phase - 2/3(freq), Frequency/1
  Amplitude - 2/1(amplitude) -> Amplitude/1
  Demux1/5 -> Hanning(Kmax+1)/3(Kmax+2)
  Demux1/1 -> Hanning(Kmax-1)/1(Kmax-2)
  Demux1/2 -> Hanning(Kmax)/1(Kmax-1), Hanning(Kmax-1)/2(Kmax-1)
  Demux1/3 -> Hanning(Kmax-1)/3(Kmax), Hanning(Kmax+1)/1(Kmax), Hanning(Kmax)/2(Kmax)
  Demux1/4 -> Hanning(Kmax+1)/2(Kmax+1), Hanning(Kmax)/3(Kmax+1)
  Hanning(Kmax+1)/1(Hanning out) -> epsilon/2(X (k max+1))
  Hanning(Kmax)/1(Hanning out) -> "delta - 1 "/1(X (k max)), Amplitude - 1/2((X k_max)), spectral leakage compensation/4(X (k max))
  epsilon/1(X (Kmax + epsilon)) -> "delta - 1 "/2(X (k max + epsilon)), spectral leakage compensation/3(X (k max + epsilon))
  epsilon/2(epsilon) -> spectral leakage compensation/5(epsilon), delta - 2/3(epsilon), "delta - 1 "/3(epsilon)
  "delta - 1 "/1(delta) -> spectral leakage compensation/2(delta), Amplitude - 1/1(delta)
  spectral leakage compensation/1(X(k max)) -> delta - 2/1(X (k max)), Complex to Magnitude-Angle2/1, Amplitude - 2/2((X k_max))
  spectral leakage compensation/2(X(k max+epsilon)) -> delta - 2/2(X (k max + epsilon))
  delta - 2/1(delta) -> Frequency - 2/1(delta), Phase - 2/2(delta), Amplitude - 2/1(delta)
  Phase - 2/1(phase) -> Phase/1
  Complex to Magnitude-Angle1/2 -> spectral leakage compensation/6(ph X(k-1))
  Complex to Magnitude-Angle1/1 -> Terminator/1
  Complex to Magnitude-Angle2/2 -> Phase - 2/1(X k_max phase)
  Complex to Magnitude-Angle2/1 -> Terminator1/1
  dT [s]/1 -> Phase - 2/4(dT [s])
  Amplitude - 1/1(amplitude) -> spectral leakage compensation/1(Amplitude)
  Hanning(Kmax-1)/1(Hanning out) -> Complex to Magnitude-Angle1/1, epsilon/1(X (k max -1))
  dF [Hz]/1 -> Frequency - 2/2(dF [Hz])

== system IEEE5BusSystemModel_std_UFLS/Subsystem3/PMU_e-IpDFT_P-class/Ia_est/mSDFT ==
  signal : Inport
  Hit : Inport  Port=2
  Delay_M : Delay  DelayLength=M  SampleTime=Ts_p
  Kmax : Subsystem
  Kmax+1 : Subsystem
  Kmax+2 : Subsystem
  Kmax-1 : Subsystem
  Kmax-2 : Subsystem
  Mux : Mux  Inputs=5
  DFT : Outport  VectorParamsAs1DForOutWhenUnconnected=off
  wires:
  Mux/1 -> DFT/1
  Kmax+2/1(X(k)) -> Mux/5
  Kmax+1/1(X(k)) -> Mux/4
  Kmax/1(X(k)) -> Mux/3
  Kmax-1/1(X(k)) -> Mux/2
  Kmax-2/1(X(k)) -> Mux/1
  signal/1 -> Kmax-2/1(x(n)), Kmax-1/1(x(n)), Kmax+2/1(x(n)), Kmax+1/1(x(n)), Kmax/1(x(n)), Delay_M/1
  Delay_M/1 -> Kmax/2(x(n-M)), Kmax+1/2(x(n-M)), Kmax+2/2(x(n-M)), Kmax-1/2(x(n-M)), Kmax-2/2(x(n-M))
  Hit/1 -> Kmax-2/3(trigger), Kmax-1/3(trigger), Kmax/3(trigger), Kmax+1/3(trigger), Kmax+2/3(trigger)

== system IEEE5BusSystemModel_std_UFLS/Subsystem3/PMU_e-IpDFT_P-class1/Ia_est/Synchrophasor estimation ==
  DFT : Inport
  dT [s] : Inport  Port=2
  dF [Hz] : Inport  Port=3
  Amplitude - 1 : Subsystem
  Amplitude - 2 : Subsystem
  Complex to Magnitude-Angle1 : ComplexToMagnitudeAngle
  Complex to Magnitude-Angle2 : ComplexToMagnitudeAngle
  Demux1 : Demux  Outputs=5
  Frequency - 2 : Subsystem
  Hanning(Kmax) : Subsystem
  Hanning(Kmax+1) : Subsystem
  Hanning(Kmax-1) : Subsystem
  Phase - 2 : Subsystem
  Terminator : Terminator
  Terminator1 : Terminator
  "delta - 1 " : Subsystem
  delta - 2 : Subsystem
  epsilon : Subsystem
  spectral leakage compensation : Subsystem
  Frequency : Outport  VectorParamsAs1DForOutWhenUnconnected=off
  Amplitude : Outport  Port=2  VectorParamsAs1DForOutWhenUnconnected=off
  Phase : Outport  Port=3  VectorParamsAs1DForOutWhenUnconnected=off
  wires:
  dF [Hz]/1 -> Frequency - 2/2(dF [Hz])
  Hanning(Kmax-1)/1(Hanning out) -> epsilon/1(X (k max -1)), Complex to Magnitude-Angle1/1
  Amplitude - 1/1(amplitude) -> spectral leakage compensation/1(Amplitude)
  dT [s]/1 -> Phase - 2/4(dT [s])
  Complex to Magnitude-Angle2/1 -> Terminator1/1
  Complex to Magnitude-Angle2/2 -> Phase - 2/1(X k_max phase)
  Complex to Magnitude-Angle1/1 -> Terminator/1
  Complex to Magnitude-Angle1/2 -> spectral leakage compensation/6(ph X(k-1))
  Phase - 2/1(phase) -> Phase/1
  delta - 2/1(delta) -> Amplitude - 2/1(delta), Phase - 2/2(delta), Frequency - 2/1(delta)
  spectral leakage compensation/2(X(k max+epsilon)) -> delta - 2/2(X (k max + epsilon))
  spectral leakage compensation/1(X(k max)) -> Amplitude - 2/2((X k_max)), Complex to Magnitude-Angle2/1, delta - 2/1(X (k max))
  "delta - 1 "/1(delta) -> Amplitude - 1/1(delta), spectral leakage compensation/2(delta)
  epsilon/2(epsilon) -> "delta - 1 "/3(epsilon), delta - 2/3(epsilon), spectral leakage compensation/5(epsilon)
  epsilon/1(X (Kmax + epsilon)) -> spectral leakage compensation/3(X (k max + epsilon)), "delta - 1 "/2(X (k max + epsilon))
  Hanning(Kmax)/1(Hanning out) -> spectral leakage compensation/4(X (k max)), Amplitude - 1/2((X k_max)), "delta - 1 "/1(X (k max))
  Hanning(Kmax+1)/1(Hanning out) -> epsilon/2(X (k max+1))
  Demux1/4 -> Hanning(Kmax)/3(Kmax+1), Hanning(Kmax+1)/2(Kmax+1)
  Demux1/3 -> Hanning(Kmax)/2(Kmax), Hanning(Kmax+1)/1(Kmax), Hanning(Kmax-1)/3(Kmax)
  Demux1/2 -> Hanning(Kmax-1)/2(Kmax-1), Hanning(Kmax)/1(Kmax-1)
  Demux1/1 -> Hanning(Kmax-1)/1(Kmax-2)
  Demux1/5 -> Hanning(Kmax+1)/3(Kmax+2)
  Amplitude - 2/1(amplitude) -> Amplitude/1
  Frequency - 2/1(frequency) -> Frequency/1, Phase - 2/3(freq)
  DFT/1 -> Demux1/1

== system IEEE5BusSystemModel_std_UFLS/Subsystem3/PMU_e-IpDFT_P-class1/Ia_est/mSDFT ==
  signal : Inport
  Hit : Inport  Port=2
  Delay_M : Delay  DelayLength=M  SampleTime=Ts_p
  Kmax : Subsystem
  Kmax+1 : Subsystem
  Kmax+2 : Subsystem
  Kmax-1 : Subsystem
  Kmax-2 : Subsystem
  Mux : Mux  Inputs=5
  DFT : Outport  VectorParamsAs1DForOutWhenUnconnected=off
  wires:
  Hit/1 -> Kmax+2/3(trigger), Kmax+1/3(trigger), Kmax/3(trigger), Kmax-1/3(trigger), Kmax-2/3(trigger)
  Delay_M/1 -> Kmax-2/2(x(n-M)), Kmax-1/2(x(n-M)), Kmax+2/2(x(n-M)), Kmax+1/2(x(n-M)), Kmax/2(x(n-M))
  signal/1 -> Delay_M/1, Kmax/1(x(n)), Kmax+1/1(x(n)), Kmax+2/1(x(n)), Kmax-1/1(x(n)), Kmax-2/1(x(n))
  Kmax-2/1(X(k)) -> Mux/1
  Kmax-1/1(X(k)) -> Mux/2
  Kmax/1(X(k)) -> Mux/3
  Kmax+1/1(X(k)) -> Mux/4
  Kmax+2/1(X(k)) -> Mux/5
  Mux/1 -> DFT/1

== system IEEE5BusSystemModel_std_UFLS/Subsystem4/PMU_e-IpDFT_P-class/Ia_est/Synchrophasor estimation ==
  DFT : Inport
  dT [s] : Inport  Port=2
  dF [Hz] : Inport  Port=3
  Amplitude - 1 : Subsystem
  Amplitude - 2 : Subsystem
  Complex to Magnitude-Angle1 : ComplexToMagnitudeAngle
  Complex to Magnitude-Angle2 : ComplexToMagnitudeAngle
  Demux1 : Demux  Outputs=5
  Frequency - 2 : Subsystem
  Hanning(Kmax) : Subsystem
  Hanning(Kmax+1) : Subsystem
  Hanning(Kmax-1) : Subsystem
  Phase - 2 : Subsystem
  Terminator : Terminator
  Terminator1 : Terminator
  "delta - 1 " : Subsystem
  delta - 2 : Subsystem
  epsilon : Subsystem
  spectral leakage compensation : Subsystem
  Frequency : Outport  VectorParamsAs1DForOutWhenUnconnected=off
  Amplitude : Outport  Port=2  VectorParamsAs1DForOutWhenUnconnected=off
  Phase : Outport  Port=3  VectorParamsAs1DForOutWhenUnconnected=off
  wires:
  dF [Hz]/1 -> Frequency - 2/2(dF [Hz])
  Hanning(Kmax-1)/1(Hanning out) -> epsilon/1(X (k max -1)), Complex to Magnitude-Angle1/1
  Amplitude - 1/1(amplitude) -> spectral leakage compensation/1(Amplitude)
  dT [s]/1 -> Phase - 2/4(dT [s])
  Complex to Magnitude-Angle2/1 -> Terminator1/1
  Complex to Magnitude-Angle2/2 -> Phase - 2/1(X k_max phase)
  Complex to Magnitude-Angle1/1 -> Terminator/1
  Complex to Magnitude-Angle1/2 -> spectral leakage compensation/6(ph X(k-1))
  Phase - 2/1(phase) -> Phase/1
  delta - 2/1(delta) -> Amplitude - 2/1(delta), Phase - 2/2(delta), Frequency - 2/1(delta)
  spectral leakage compensation/2(X(k max+epsilon)) -> delta - 2/2(X (k max + epsilon))
  spectral leakage compensation/1(X(k max)) -> Amplitude - 2/2((X k_max)), Complex to Magnitude-Angle2/1, delta - 2/1(X (k max))
  "delta - 1 "/1(delta) -> Amplitude - 1/1(delta), spectral leakage compensation/2(delta)
  epsilon/2(epsilon) -> "delta - 1 "/3(epsilon), delta - 2/3(epsilon), spectral leakage compensation/5(epsilon)
  epsilon/1(X (Kmax + epsilon)) -> spectral leakage compensation/3(X (k max + epsilon)), "delta - 1 "/2(X (k max + epsilon))
  Hanning(Kmax)/1(Hanning out) -> spectral leakage compensation/4(X (k max)), Amplitude - 1/2((X k_max)), "delta - 1 "/1(X (k max))
  Hanning(Kmax+1)/1(Hanning out) -> epsilon/2(X (k max+1))
  Demux1/4 -> Hanning(Kmax)/3(Kmax+1), Hanning(Kmax+1)/2(Kmax+1)
  Demux1/3 -> Hanning(Kmax)/2(Kmax), Hanning(Kmax+1)/1(Kmax), Hanning(Kmax-1)/3(Kmax)
  Demux1/2 -> Hanning(Kmax-1)/2(Kmax-1), Hanning(Kmax)/1(Kmax-1)
  Demux1/1 -> Hanning(Kmax-1)/1(Kmax-2)
  Demux1/5 -> Hanning(Kmax+1)/3(Kmax+2)
  Amplitude - 2/1(amplitude) -> Amplitude/1
  Frequency - 2/1(frequency) -> Frequency/1, Phase - 2/3(freq)
  DFT/1 -> Demux1/1

== system IEEE5BusSystemModel_std_UFLS/Subsystem4/PMU_e-IpDFT_P-class/Ia_est/mSDFT ==
  signal : Inport
  Hit : Inport  Port=2
  Delay_M : Delay  DelayLength=M  SampleTime=Ts_p
  Kmax : Subsystem
  Kmax+1 : Subsystem
  Kmax+2 : Subsystem
  Kmax-1 : Subsystem
  Kmax-2 : Subsystem
  Mux : Mux  Inputs=5
  DFT : Outport  VectorParamsAs1DForOutWhenUnconnected=off
  wires:
  Hit/1 -> Kmax+2/3(trigger), Kmax+1/3(trigger), Kmax/3(trigger), Kmax-1/3(trigger), Kmax-2/3(trigger)
  Delay_M/1 -> Kmax-2/2(x(n-M)), Kmax-1/2(x(n-M)), Kmax+2/2(x(n-M)), Kmax+1/2(x(n-M)), Kmax/2(x(n-M))
  signal/1 -> Delay_M/1, Kmax/1(x(n)), Kmax+1/1(x(n)), Kmax+2/1(x(n)), Kmax-1/1(x(n)), Kmax-2/1(x(n))
  Kmax-2/1(X(k)) -> Mux/1
  Kmax-1/1(X(k)) -> Mux/2
  Kmax/1(X(k)) -> Mux/3
  Kmax+1/1(X(k)) -> Mux/4
  Kmax+2/1(X(k)) -> Mux/5
  Mux/1 -> DFT/1

== system IEEE5BusSystemModel_std_UFLS/Subsystem4/PMU_e-IpDFT_P-class1/Ia_est/Synchrophasor estimation ==
  DFT : Inport
  dT [s] : Inport  Port=2
  dF [Hz] : Inport  Port=3
  Amplitude - 1 : Subsystem
  Amplitude - 2 : Subsystem
  Complex to Magnitude-Angle1 : ComplexToMagnitudeAngle
  Complex to Magnitude-Angle2 : ComplexToMagnitudeAngle
  Demux1 : Demux  Outputs=5
  Frequency - 2 : Subsystem
  Hanning(Kmax) : Subsystem
  Hanning(Kmax+1) : Subsystem
  Hanning(Kmax-1) : Subsystem
  Phase - 2 : Subsystem
  Terminator : Terminator
  Terminator1 : Terminator
  "delta - 1 " : Subsystem
  delta - 2 : Subsystem
  epsilon : Subsystem
  spectral leakage compensation : Subsystem
  Frequency : Outport  VectorParamsAs1DForOutWhenUnconnected=off
  Amplitude : Outport  Port=2  VectorParamsAs1DForOutWhenUnconnected=off
  Phase : Outport  Port=3  VectorParamsAs1DForOutWhenUnconnected=off
  wires:
  DFT/1 -> Demux1/1
  Frequency - 2/1(frequency) -> Phase - 2/3(freq), Frequency/1
  Amplitude - 2/1(amplitude) -> Amplitude/1
  Demux1/5 -> Hanning(Kmax+1)/3(Kmax+2)
  Demux1/1 -> Hanning(Kmax-1)/1(Kmax-2)
  Demux1/2 -> Hanning(Kmax)/1(Kmax-1), Hanning(Kmax-1)/2(Kmax-1)
  Demux1/3 -> Hanning(Kmax-1)/3(Kmax), Hanning(Kmax+1)/1(Kmax), Hanning(Kmax)/2(Kmax)
  Demux1/4 -> Hanning(Kmax+1)/2(Kmax+1), Hanning(Kmax)/3(Kmax+1)
  Hanning(Kmax+1)/1(Hanning out) -> epsilon/2(X (k max+1))
  Hanning(Kmax)/1(Hanning out) -> "delta - 1 "/1(X (k max)), Amplitude - 1/2((X k_max)), spectral leakage compensation/4(X (k max))
  epsilon/1(X (Kmax + epsilon)) -> "delta - 1 "/2(X (k max + epsilon)), spectral leakage compensation/3(X (k max + epsilon))
  epsilon/2(epsilon) -> spectral leakage compensation/5(epsilon), delta - 2/3(epsilon), "delta - 1 "/3(epsilon)
  "delta - 1 "/1(delta) -> spectral leakage compensation/2(delta), Amplitude - 1/1(delta)
  spectral leakage compensation/1(X(k max)) -> delta - 2/1(X (k max)), Complex to Magnitude-Angle2/1, Amplitude - 2/2((X k_max))
  spectral leakage compensation/2(X(k max+epsilon)) -> delta - 2/2(X (k max + epsilon))
  delta - 2/1(delta) -> Frequency - 2/1(delta), Phase - 2/2(delta), Amplitude - 2/1(delta)
  Phase - 2/1(phase) -> Phase/1
  Complex to Magnitude-Angle1/2 -> spectral leakage compensation/6(ph X(k-1))
  Complex to Magnitude-Angle1/1 -> Terminator/1
  Complex to Magnitude-Angle2/2 -> Phase - 2/1(X k_max phase)
  Complex to Magnitude-Angle2/1 -> Terminator1/1
  dT [s]/1 -> Phase - 2/4(dT [s])
  Amplitude - 1/1(amplitude) -> spectral leakage compensation/1(Amplitude)
  Hanning(Kmax-1)/1(Hanning out) -> Complex to Magnitude-Angle1/1, epsilon/1(X (k max -1))
  dF [Hz]/1 -> Frequency - 2/2(dF [Hz])
